simulink model "trajectory_m"  (R2023b)
settings: Solver=ode8  StartTime=0.0  StopTime=T  FixedStep=10e-3  RelTol=1e-3
values from neighbouring files (symbols this model uses):
  K = obj.P*(obj.Ad(obj.X)')*(H')*S_inv    [riekf_SE3.m]    (also in riekf_localization_SE3.m = 1.13333333333)
  Kp = 1.5    [riekf_localization_SE3.m]
  V0M = V0M/sqrt(V0M*V0M')    [riekf_localization_SE3.m]
  V_M = 15    [riekf_localization_SE3.m]
  V_T = 17    [riekf_localization_SE3.m]
  X0M = [0 0 0]    [riekf_localization_SE3.m]
  X0T = [0; 0 ;5]    [riekf_localization_SE3.m]
libraries: matrix_library x7, shared6dof x1, aerolibanim x1
settings Model: Creator=jacek  LastModifiedBy=Jacek
settings SolverCC: MaxConsecutiveMinStep=3
settings DebuggingCC: UnconnectedInputMsg=warning  UnconnectedOutputMsg=warning  UnconnectedLineMsg=warning
settings ModelReferenceCC: EnableRefExpFcnMdlSchedulingChecks=on
settings RTWCC: DLArmComputeVersion=19.05

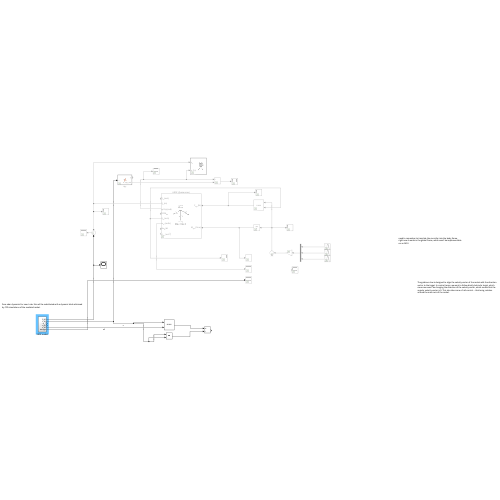
[thumbnail: Simulink's stored preview of the top-level diagram]
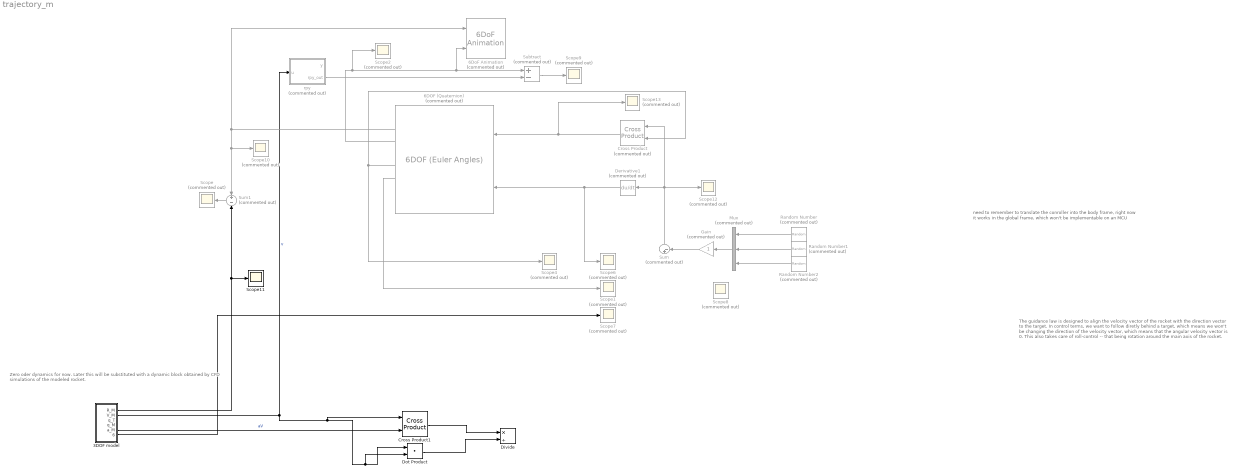
== system trajectory_m ==
  note: need to remember to translate the conroller into the body frame,
      | right now it works in the global frame, which won't be implementable
      | on an MCU
  note: The guidance law is designed to align the velocity vector of the rocket with the direction vector to the target. In control terms, we want to follow diretly behind a target, which means we won't be changing the direction of the velocity vector, which means that the angular velocity vector is 0. This also takes care of roll-control -- that being rotation around the main axis of the rocket.
  note: Zero oder dynamics for now. Later this will be substituted with a dynamic block obtained by CFD simulations of the modeled rocket.
  3DOF model : Subsystem
  6DOF (Quaternion) : shared6dof/6DOF (Euler Angles)  Commented=on  units=Metric (MKS)  mtype=Fixed  rep=Quaternion  xme_0=X0M  Vm_0=[0,0,1]  eul_0=rpy  pm_0=omega_0  mass_0=1  mass_e=0.5  mass_f=2.0  inertia=eye(3)  inertia_e=eye(3)  inertia_f=2*eye(3)  k_quat=10  vre_flag=on  abi_flag=off  aMode=0  xme_statename=''  Vm_statename=''  eul_statename=''  quat_statename=''  pm_statename=''  mass_statename=''
  6DoF Animation : aerolibanim/6DoF Animation  Commented=on  u1=[0 4000 -2000 2000 -5000 -3000]  u2=0.1  u3=1.0  u4=[0 0 0]  u5=Fixed position  u6=[10 10 0]  u7=10  u8=on
  Cross Product : matrix_library/Cross Product  Commented=on
  Cross Product1 : matrix_library/Cross Product
  Derivative1 : Derivative  Commented=on
  Divide : Product  Inputs=*/
  Dot Product : DotProduct  OutDataTypeStr=Inherit: Inherit via internal rule
  Gain : Gain  Commented=on
  Mux : Mux  Commented=on  Inputs=3
  Random Number : RandomNumber  Commented=on  Variance=0.0017  Seed=1  SampleTime=0.1
  Random Number1 : RandomNumber  Commented=on  Variance=0.0017  Seed=17  SampleTime=0.1
  Random Number2 : RandomNumber  Commented=on  Variance=0.0017  Seed=37  SampleTime=0.1
  Scope{,1..2,4,6..10,12..13} (11 alike) : Scope  Commented=on
  Scope11 : Scope
  Subtract : Sum  Commented=on  Inputs=+-
  Sum : Sum  Commented=on  Inputs=|+-
  Sum1 : Sum  Commented=on  Inputs=+-
  rpy : MATLAB Function  Commented=on  TreatAsAtomicUnit=on
  wires:
  Sum1/1 -> Scope/1
  6DOF (Quaternion)/5 -> Cross Product/2, Scope4/1
  6DOF (Quaternion)/6 -> Scope1/1
  Derivative1/1 -> 6DOF (Quaternion)/2, Scope6/1
  rpy/2(rpy_out) -> Subtract/2
  3DOF model/1(R_M) -> Scope11/1, Sum1/2
  3DOF model/2(V_M) -> Dot Product/1, Dot Product/2, Cross Product1/1, rpy/1(u)  "v"
  3DOF model/5(a_M) -> Cross Product1/2  "aV"
  Cross Product1/1 -> Divide/1
  Dot Product/1 -> Divide/2
  3DOF model/6(omega) -> Scope7/1
  Subtract/1 -> Scope9/1
  Cross Product/1 -> 6DOF (Quaternion)/1, Scope13/1
  6DOF (Quaternion)/2 -> Scope10/1, Sum1/1, 6DoF Animation/1
  Sum/1 -> Scope12/1, Derivative1/1, Cross Product/1
  Random Number/1 -> Mux/1
  Random Number1/1 -> Mux/2
  Random Number2/1 -> Mux/3
  Mux/1 -> Gain/1
  Gain/1 -> Sum/2
  6DOF (Quaternion)/3 -> Scope2/1, 6DoF Animation/2, Subtract/1

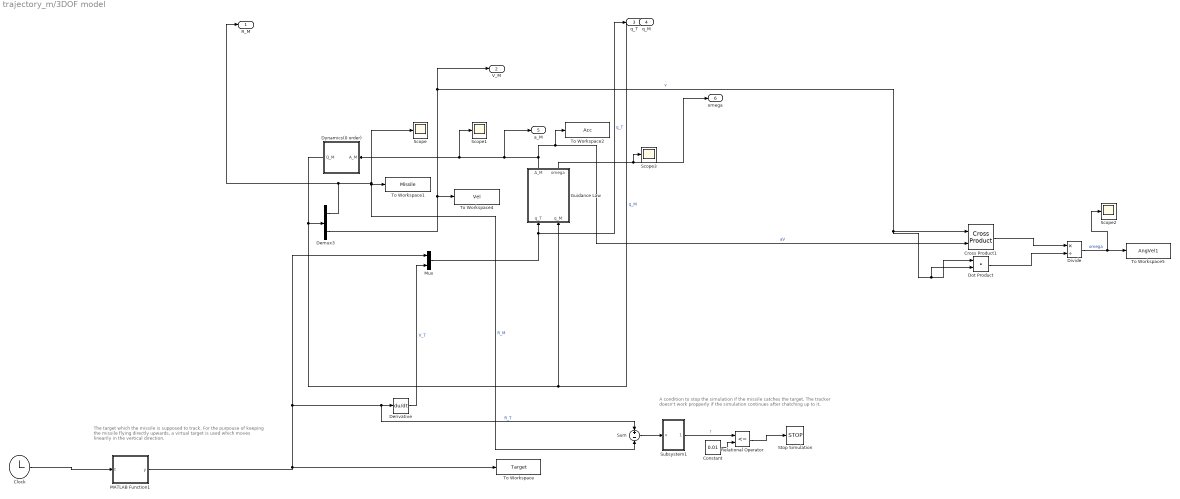
== system trajectory_m/3DOF model ==
  note: A condition to stop the simulation if the missile catches the target.
      | The tracker doesn't work propperly if the simulation continues after chatching
      | up to it.
  note: The target which the missile is supposed to track.
      | For the purpouse of keeping the missile flying directly upwards, a virtual
      | target is used which moves linearily in the vertical direction.
  Clock : Clock
  Constant : Constant  Value=0.01
  Cross Product1 : matrix_library/Cross Product
  Demux3 : Demux  Outputs=[3,3]
  Derivative : Derivative
  Divide : Product  Inputs=*/
  Dot Product : DotProduct  OutDataTypeStr=Inherit: Inherit via internal rule
  Dynamics(0 order) : Subsystem
  Guidance Law : Subsystem
  MATLAB Function1 : MATLAB Function  TreatAsAtomicUnit=on
  Mux : Mux  Inputs=2
  Relational Operator : RelationalOperator  Operator=<=  OutDataTypeStr=boolean  RndMeth=Simplest  InputSameDT=off
  Scope{,1..3} (4 alike) : Scope
  Stop Simulation : Stop
  Subsystem1 : Subsystem
  Sum : Sum  Inputs=+-
  To Workspace : ToWorkspace  VariableName=Target  SaveFormat=Timeseries  SampleTime=-1
  To Workspace1 : ToWorkspace  VariableName=Missile  SaveFormat=Timeseries  SampleTime=-1
  To Workspace2 : ToWorkspace  VariableName=Acc  SaveFormat=Timeseries  SampleTime=-1
  To Workspace4 : ToWorkspace  VariableName=Vel  SaveFormat=Timeseries  SampleTime=-1
  To Workspace5 : ToWorkspace  VariableName=AngVel1  SaveFormat=Timeseries  SampleTime=-1
  R_M : Outport
  V_M : Outport  Port=2
  q_T : Outport  Port=3
  q_M : Outport  Port=4
  a_M : Outport  Port=5
  omega : Outport  Port=6
  wires:
  Constant/1 -> Relational Operator/2
  Relational Operator/1 -> Stop Simulation/1
  Sum/1 -> Subsystem1/1(v)
  Clock/1 -> MATLAB Function1/1(t)
  Mux/1 -> q_T/1, Guidance Law/1(q_T)  "q_T"
  MATLAB Function1/1(y) -> Sum/1, Derivative/1, Mux/1, To Workspace/1  "R_T"
  Derivative/1 -> Mux/2  "V_T"
  Demux3/1 -> R_M/1, Sum/2, To Workspace1/1, Scope/1  "R_M"
  Guidance Law/2(omega) -> Scope3/1, omega/1
  Subsystem1/1(norm) -> Relational Operator/1  "r"
  Dynamics(0 order)/1(Q_M) -> q_M/1, Guidance Law/2(q_M), Demux3/1  "q_M"
  Dot Product/1 -> Divide/2
  Demux3/2 -> Dot Product/1, Dot Product/2, Cross Product1/1, V_M/1, To Workspace4/1  "v"
  Guidance Law/1(A_M) -> To Workspace2/1, Cross Product1/2, a_M/1, Scope1/1, Dynamics(0 order)/1(A_M)  "aV"
  Cross Product1/1 -> Divide/1
  Divide/1 -> Scope2/1, To Workspace5/1  "omega"

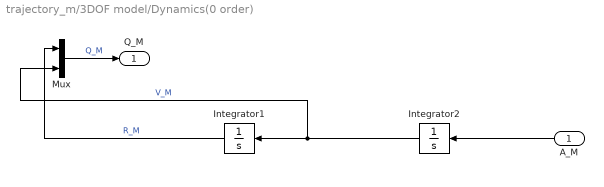
== system trajectory_m/3DOF model/Dynamics(0 order) ==
  A_M : Inport
  Integrator1 : Integrator  InitialCondition=X0M
  Integrator2 : Integrator  InitialCondition=V0M*V_M
  Mux : Mux  Inputs=2
  Q_M : Outport
  wires:
  Integrator1/1 -> Mux/1  "R_M"
  Integrator2/1 -> Integrator1/1, Mux/2  "V_M"
  A_M/1 -> Integrator2/1
  Mux/1 -> Q_M/1  "Q_M"

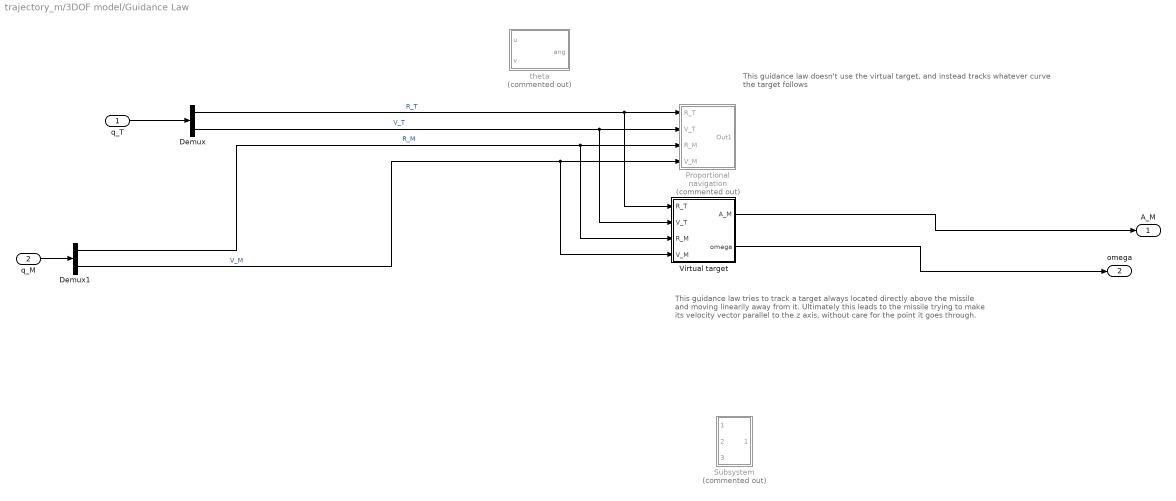
== system trajectory_m/3DOF model/Guidance Law ==
  note: This guidance law tries to track a target always located directly above
      | the missile and moving linearily away from it. Ultimately this leads to the
      | missile trying to make its velocity vector parallel to the z axis, without care for
      | the point it goes through.
  note: This guidance law doesn't use the virtual target, and instead tracks whatever
      | curve the target follows
  q_T : Inport
  q_M : Inport  Port=2
  Demux : Demux  Outputs=[3,3]
  Demux1 : Demux  Outputs=[3,3]
  Proportional navigation : Subsystem  Commented=on
  Subsystem : Subsystem  Commented=on
  Virtual target : Subsystem
  theta : MATLAB Function  Commented=on  TreatAsAtomicUnit=on
  A_M : Outport  PortDimensions=3
  omega : Outport  Port=2  PortDimensions=3
  wires:
  q_T/1 -> Demux/1
  q_M/1 -> Demux1/1
  Demux/1 -> Virtual target/1(R_T), Proportional navigation/1(R_T)  "R_T"
  Demux/2 -> Virtual target/2(V_T), Proportional navigation/2(V_T)  "V_T"
  Demux1/1 -> Virtual target/3(R_M), Proportional navigation/3(R_M)  "R_M"
  Demux1/2 -> Virtual target/4(V_M), Proportional navigation/4(V_M)  "V_M"
  Virtual target/1(A_M) -> A_M/1
  Virtual target/2(omega) -> omega/1

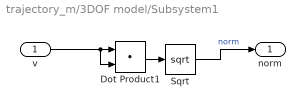
== system trajectory_m/3DOF model/Subsystem1 ==
  v : Inport
  Dot Product1 : DotProduct  OutDataTypeStr=Inherit: Inherit via internal rule
  Sqrt : Sqrt
  norm : Outport
  wires:
  Dot Product1/1 -> Sqrt/1
  v/1 -> Dot Product1/2, Dot Product1/1
  Sqrt/1 -> norm/1  "norm"

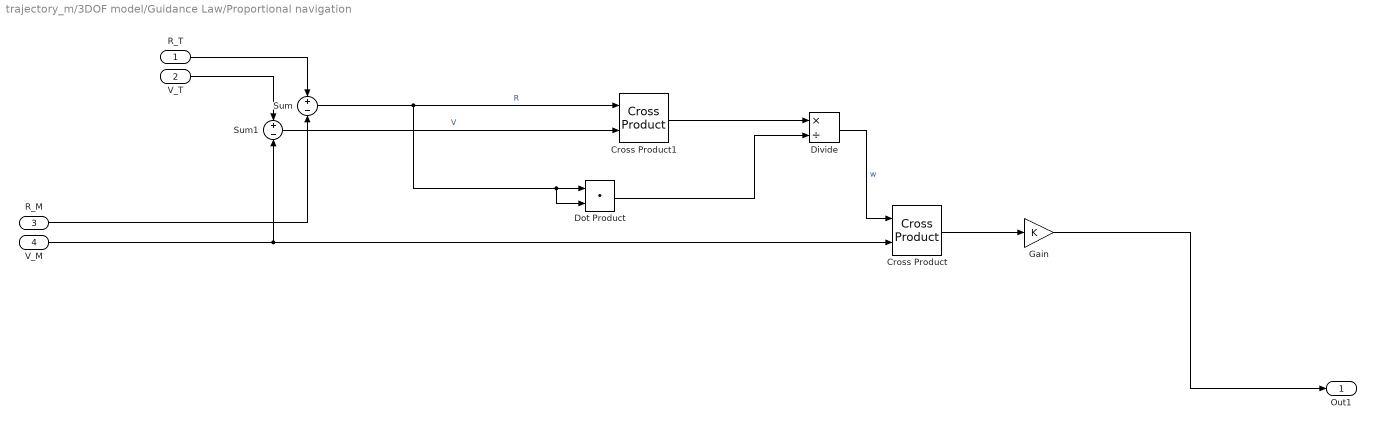
== system trajectory_m/3DOF model/Guidance Law/Proportional navigation ==
  R_T : Inport
  V_T : Inport  Port=2
  R_M : Inport  Port=3
  V_M : Inport  Port=4
  Cross Product : matrix_library/Cross Product
  Cross Product1 : matrix_library/Cross Product
  Divide : Product  Inputs=*/
  Dot Product : DotProduct  OutDataTypeStr=Inherit: Inherit via internal rule
  Gain : Gain  Gain=K
  Sum : Sum  Inputs=+-
  Sum1 : Sum  Inputs=+-
  Out1 : Outport
  wires:
  R_T/1 -> Sum/1
  V_T/1 -> Sum1/1
  Gain/1 -> Out1/1
  Cross Product/1 -> Gain/1
  Dot Product/1 -> Divide/2
  Divide/1 -> Cross Product/1  "w"
  V_M/1 -> Sum1/2, Cross Product/2
  Sum/1 -> Cross Product1/1, Dot Product/2, Dot Product/1  "R"
  Cross Product1/1 -> Divide/1
  Sum1/1 -> Cross Product1/2  "V"
  R_M/1 -> Sum/2

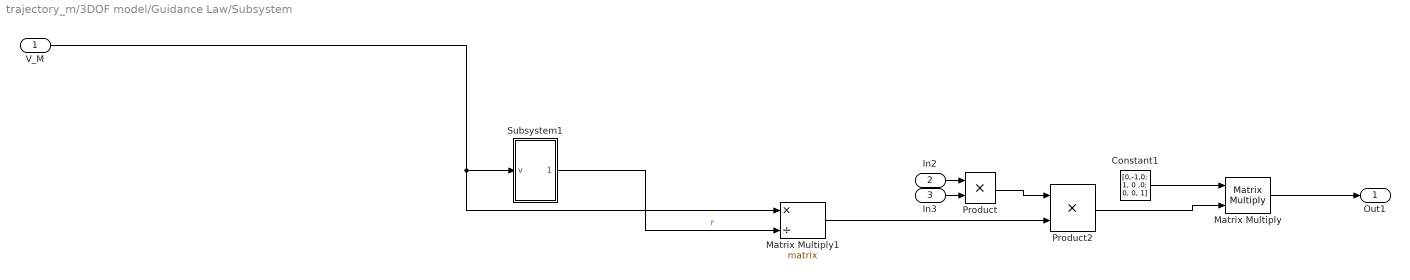
== system trajectory_m/3DOF model/Guidance Law/Subsystem ==
  V_M : Inport
  In2 : Inport  Port=2
  In3 : Inport  Port=3
  Constant1 : Constant  Value=[0,-1,0; 1, 0 ,0; 0, 0, 1]
  Matrix Multiply : Product  Multiplication=Matrix(*)
  Matrix Multiply1 : Product  Inputs=*/  Multiplication=Matrix(*)
  Product : Product
  Product2 : Product
  Subsystem1 : Subsystem
  Out1 : Outport
  wires:
  Product/1 -> Product2/1
  Constant1/1 -> Matrix Multiply/1
  Product2/1 -> Matrix Multiply/2
  V_M/1 -> Matrix Multiply1/1, Subsystem1/1(v)
  In2/1 -> Product/1
  Matrix Multiply/1 -> Out1/1
  Subsystem1/1(norm) -> Matrix Multiply1/2  "r"
  In3/1 -> Product/2
  Matrix Multiply1/1 -> Product2/2

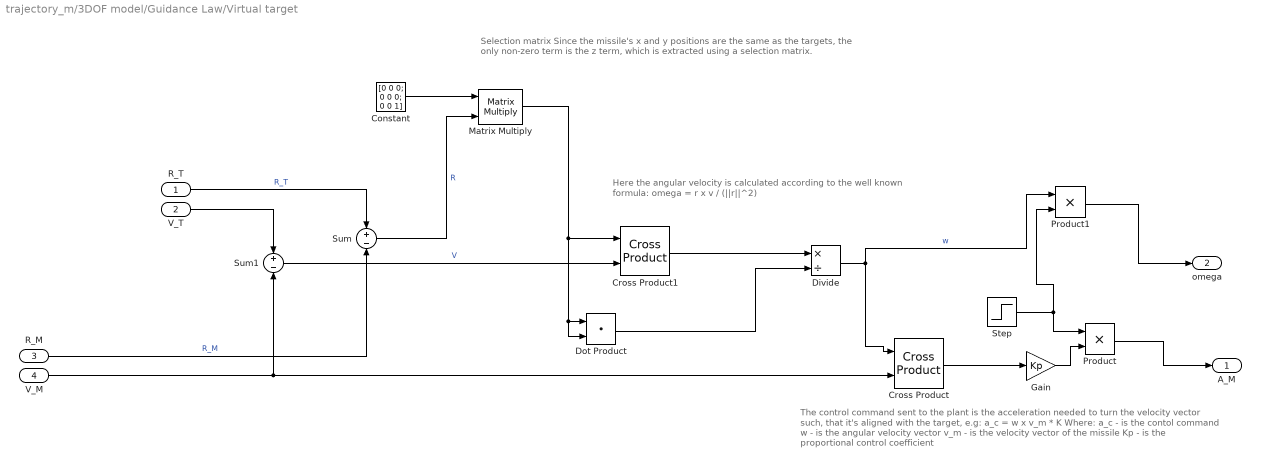
== system trajectory_m/3DOF model/Guidance Law/Virtual target ==
  note: The control command sent to the plant  is the acceleration needed to turn the velocity vector such, that it's aligned with the target, e.g:
      |
      | a_c = w x v_m * K
      |
      | Where:
      | a_c    -  is the contol command
      | w       -  is the angular velocity vector
      | v_m   - is the velocity vector of the missile
      | Kp       - is the proportional control coefficient
  note: Here the angular velocity is calculated according to the well known
      | formula: omega = r x v / (||r||^2)
  note: Selection matrix
      | Since the missile's x and y positions are the same as the targets,
      | the only non-zero term is the z term, which is extracted using a selection matrix.
  R_T : Inport
  V_T : Inport  Port=2
  R_M : Inport  Port=3
  V_M : Inport  Port=4
  Constant : Constant  Value=[0 0 0; 0 0 0; 0 0 1]
  Cross Product : matrix_library/Cross Product
  Cross Product1 : matrix_library/Cross Product
  Divide : Product  Inputs=*/
  Dot Product : DotProduct  OutDataTypeStr=Inherit: Inherit via internal rule
  Gain : Gain  Gain=Kp
  Matrix Multiply : Product  Inputs=**  Multiplication=Matrix(*)
  Product : Product
  Product1 : Product
  Step : Step  Time=15  SampleTime=0
  Sum : Sum  Inputs=+-
  Sum1 : Sum  Inputs=+-
  A_M : Outport
  omega : Outport  Port=2
  wires:
  R_T/1 -> Sum/1  "R_T"
  V_T/1 -> Sum1/1
  Cross Product/1 -> Gain/1
  Dot Product/1 -> Divide/2
  V_M/1 -> Sum1/2, Cross Product/2
  Sum/1 -> Matrix Multiply/2  "R"
  Cross Product1/1 -> Divide/1
  Sum1/1 -> Cross Product1/2  "V"
  R_M/1 -> Sum/2  "R_M"
  Constant/1 -> Matrix Multiply/1
  Matrix Multiply/1 -> Dot Product/2, Dot Product/1, Cross Product1/1
  Divide/1 -> Product1/1, Cross Product/1  "w"
  Gain/1 -> Product/2
  Product/1 -> A_M/1
  Step/1 -> Product/1, Product1/2
  Product1/1 -> omega/1

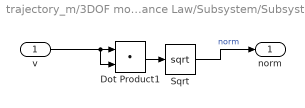
== system trajectory_m/3DOF model/Guidance Law/Subsystem/Subsystem1 ==
  v : Inport
  Dot Product1 : DotProduct  OutDataTypeStr=Inherit: Inherit via internal rule
  Sqrt : Sqrt
  norm : Outport
  wires:
  Dot Product1/1 -> Sqrt/1
  v/1 -> Dot Product1/2, Dot Product1/1
  Sqrt/1 -> norm/1  "norm"

== matlab function trajectory_m/3DOF model/MATLAB Function1 ==
  data: t input double size=1; y output double; X0T parameter; K parameter; V_T parameter
function y  = target(t,X0T,K,V_T)
y = [0  ; 0  ; V_T*t]+X0T;
%y = [0  ; 0  ; K*t]+X0T;

end

== matlab function trajectory_m/rpy ==
  data: u input; y output; rpy_out output
function [y, rpy_out] = fcn(u)


roll = -atan2(u(2),u(3));
pitch = asin(u(1));
yaw = 0;


Rx = [1 0 0 ; 0 cos(roll) -sin(roll);0 sin(roll) cos(roll)];
Ry = [cos(pitch) 0 sin(pitch); 0 1 0;-sin(pitch) 0 cos(pitch) ];
Rz = [cos(yaw) -sin(yaw) 0 ;sin(yaw) cos(yaw) 0 ; 0 0 1];


y = Rx*Ry*Rz;
rpy_out = [roll, pitch, yaw];

== matlab function trajectory_m/3DOF model/Guidance Law/theta ==
  data: u input; ang output; v input
function ang = fcn(u,v)

ang = atan2(norm(cross(u,v)),dot(u,v));
